simulink model "MK_elem"  (R2025b)
settings: Solver=VariableStepAuto  StartTime=0.0  StopTime=10.0  RelTol=1e-3
settings Model: Creator=d.alazard  LastModifiedBy=andre
settings SolverCC: AlgebraicLoopSolver=TrustRegion
settings DebuggingCC: UnconnectedInputMsg=warning  UnconnectedOutputMsg=warning  UnconnectedLineMsg=warning
settings ModelReferenceCC: EnableRefExpFcnMdlSchedulingChecks=on
settings RTWCC: GPUComputeCapability=3.5

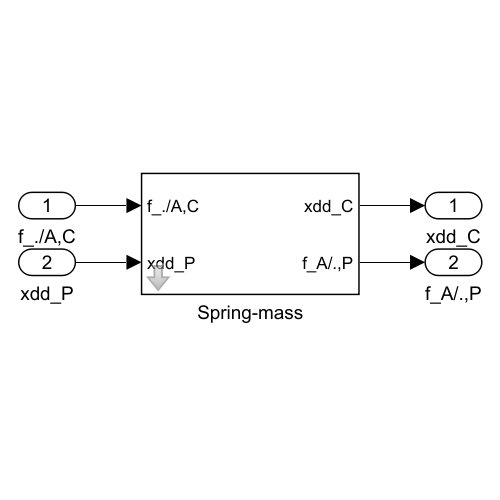
[thumbnail: Simulink's stored preview of the top-level diagram]
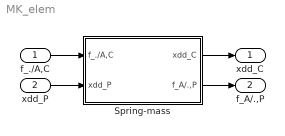
== system MK_elem ==
  f_./A,C : Inport
  xdd_P : Inport  Port=2
  Spring-mass : Subsystem  mask(Spring mass system){k=1, m_P=2, m_C=3}
      mask prompts: k "stiffness k (N/m)"; m_P "mass m_P (Kg)"; m_C "mass m_C (Kg)"
      mask help: TITOP model of the spring-mass system
  xdd_C : Outport
  f_A/.,P : Outport  Port=2
  wires:
  f_./A,C/1 -> Spring-mass/1(f_./A,C)
  xdd_P/1 -> Spring-mass/2(xdd_P)
  Spring-mass/1(xdd_C) -> xdd_C/1
  Spring-mass/2(f_A/.,P) -> f_A/.,P/1

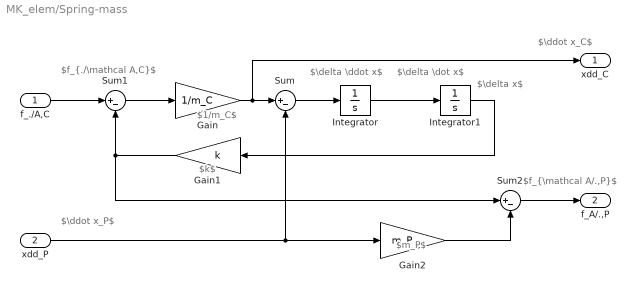
== system MK_elem/Spring-mass ==
  note: $\delta x$
  note: $\delta \dot x$
  note: $\delta \ddot x$
  note: $\ddot x_P$
  note: $\ddot x_C$
  note: $f_{\mathcal A/.,P}$
  note: $f_{./\mathcal A,C}$
  note: $1/m_C$
  note: $k$
  note: $m_P$
  f_./A,C : Inport
  xdd_P : Inport  Port=2
  Gain : Gain  Gain=1/m_C
  Gain1 : Gain  Gain=k
  Gain2 : Gain  Gain=m_P
  Integrator : Integrator
  Integrator1 : Integrator
  Sum : Sum  Inputs=|+-
  Sum1 : Sum  Inputs=|+-
  Sum2 : Sum  Inputs=|+-
  xdd_C : Outport
  f_A/.,P : Outport  Port=2
  wires:
  Sum2/1 -> f_A/.,P/1
  Integrator/1 -> Integrator1/1
  Gain1/1 -> Sum2/1, Sum1/2
  Sum1/1 -> Gain/1
  Sum/1 -> Integrator/1
  xdd_P/1 -> Gain2/1, Sum/2
  Integrator1/1 -> Gain1/1
  Gain/1 -> xdd_C/1, Sum/1
  Gain2/1 -> Sum2/2
  f_./A,C/1 -> Sum1/1
